simulink model "LAB1_Manchester"  (R2020a)
settings: Solver=VariableStepAuto  StartTime=0.0  StopTime=10.0  RelTol=1e-3
libraries: commrandsrc3 x1
settings Model: Creator=Sameer  LastModifiedBy=Sameer

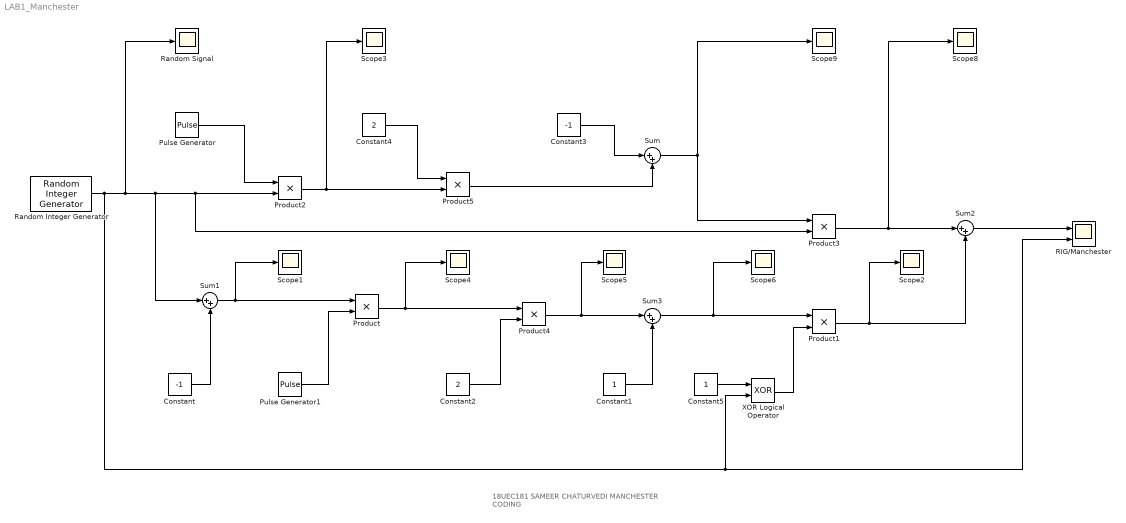
== system LAB1_Manchester ==
  note: 18UEC181
      | SAMEER CHATURVEDI
      | MANCHESTER CODING
  Constant : Constant  Value=-1
  Constant1 : Constant
  Constant2 : Constant  Value=2
  Constant3 : Constant  Value=-1
  Constant4 : Constant  Value=2
  Constant5 : Constant
  Product{,1..5} (6 alike) : Product
  Pulse Generator : DiscretePulseGenerator  PulseType=Time based  Period=1  PulseWidth=50
  Pulse Generator1 : DiscretePulseGenerator  PulseType=Time based  Period=1  PulseWidth=50
  RIG/Manchester : Scope  NumInputPorts=2
  Random Integer Generator : commrandsrc3/Random Integer Generator  SetSize=2  SeedSource=Auto  Seed=0  SampleTime=1  SamplesPerFrame=1  OutputDataType=double  SimulateUsing=Interpreted execution
  Random Signal : Scope
  Scope{1..6,8..9} (8 alike) : Scope
  Sum{,1..3} (4 alike) : Sum  Inputs=|++
  XOR Logical Operator : Logic  Operator=XOR  AllPortsSameDT=off  OutDataTypeStr=boolean
  wires:
  Random Integer Generator/1 -> XOR Logical Operator/2, RIG/Manchester/2, Random Signal/1, Sum1/1, Product3/2, Product2/2
  Pulse Generator/1 -> Product2/1
  Constant/1 -> Sum1/2
  Sum1/1 -> Product/1, Scope1/1
  Product2/1 -> Scope3/1, Product5/2
  Constant4/1 -> Product5/1
  Pulse Generator1/1 -> Product/2
  Product/1 -> Product4/1, Scope4/1
  Constant2/1 -> Product4/2
  Product4/1 -> Sum3/1, Scope5/1
  Product5/1 -> Sum/2
  Constant3/1 -> Sum/1
  Constant1/1 -> Sum3/2
  Sum3/1 -> Product1/1, Scope6/1
  Product1/1 -> Scope2/1, Sum2/2
  Sum/1 -> Product3/1, Scope9/1
  Product3/1 -> Scope8/1, Sum2/1
  Sum2/1 -> RIG/Manchester/1
  XOR Logical Operator/1 -> Product1/2
  Constant5/1 -> XOR Logical Operator/1
